simulink model "MovimientoArmonicoAmortiguado"  (R2024b)
settings: Solver=ode4  StartTime=0.0  StopTime=100.0  FixedStep=0.01  RelTol=1e-3
settings Model: Creator=Miguel  LastModifiedBy=Miguel

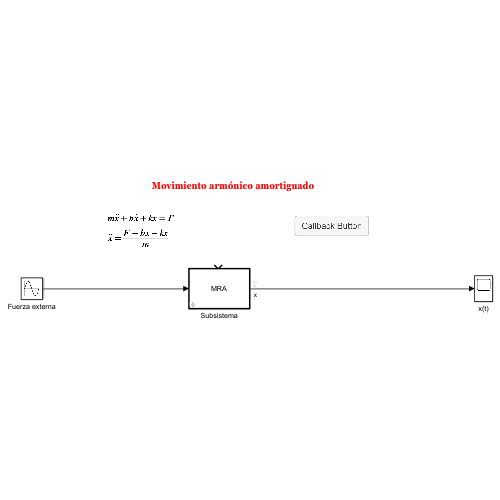
[thumbnail: Simulink's stored preview of the top-level diagram]
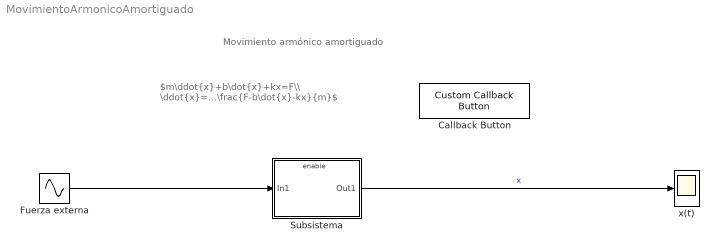
== system MovimientoArmonicoAmortiguado ==
  note: $m\ddot{x}+b\dot{x}+kx=F\\ \ddot{x}=\frac{F-b\dot{x}-kx}{m}$
  note: Movimiento armónico amortiguado
  Callback Button : CustomCallbackButton  Configuration="{\"components\":[{\"name\":\"BackgroundImageComponent\",\"settings\":{\"image\":{\"size\":[0,0],\"src\":\"default\",\"srcOrientation\":\"Right\"},\"position\":[0,0,1,1]}},{\"name\":\"ButtonStateComponent\",\"settings\":{\"buttonType\":\"momentary\",\"clickFcn\":\"close all\\nx = out.posicion;\\nv = out.velocidad;\\nn = length(x(1,:));\\n\\nplot(x(:,2),v(:,2),'LineWidth',3)\\nhold on\\n\\nfor k=3:n\\n    plot(x(:,k),v(:,k),'LineWidth',3)\\nend\\n\\nxlabel('$x$','Interpreter','latex','FontSize',14)\\nxlabel('$\\\\dot{x}$','Interpreter','latex','FontSize',14)\\ngrid on\\nhold off\",\"onValue\":1,\"position\":[0,0,1,1],\"pressDelay\":\"500\",\"pressFcn\":\"\",\"repeatInterval\":\"0\",\"states\":[{\"horizontalAlignment\":\"center\",\"image\":{\"position\":[0,0,1,1],\"size\":[1,1],\"src\":\"default\",\"srcOrientation\":\"Right\"},\"label\":{\"color\":[0.01176470588,0.01176470588,0.01176470588,1],\"icon\":{\"size\":[0,0],\"src\":\"default\",\"srcOrientation\":\"Right\"},\"iconOffset\":0,\"iconPlacement\":\"left\",\"opacity\":1,\"show\":true,\"text\":{\"content\":\"Callback Button\",\"font\":\"Helvetica\"}},\"labelOffset\":[0,0],\"verticalAlignment\":\"middle\"},{\"horizontalAlignment\":\"center\",\"image\":{\"position\":[0,0,1,1],\"size\":[1,1],\"src\":\"default\",\"srcOrientation\":\"Right\"},\"label\":{\"color\":[0.01176470588,0.01176470588,0.01176470588,1],\"icon\":{\"size\":[0,0],\"src\":\"default\",\"srcOrientation\":\"Right\"},\"iconOffset\":0,\"iconPlacement\":\"left\",\"opacity\":1,\"show\":true,\"text\":{\"content\":\"Callback Button\",\"font\":\"Helvetica\"}},\"labelOffset\":[0,0],\"verticalAlignment\":\"middle\"},{\"horizontalAlignment\":\"center\",\"image\":{\"position\":[0,0,1,1],\"size\":[1,1],\"src\":\"default\",\"srcOrientation\":\"Right\"},\"label\":{\"color\":[0.01176470588,0.01176470588,0.01176470588,1],\"icon\":{\"size\":[0,0],\"src\":\"default\",\"srcOrientation\":\"Right\"},\"iconOffset\":0,\"iconPlacement\":\"left\",\"opacity\":1,\"show\":true,\"text\":{\"content\":\"Callback Button\",\"font\":\"Helvetica\"}},\"labelOffset\":[0,0],\"verticalAlignment\":\"middle\"},{\"horizontalAlignment\":\"center\",\"image\":{\"position\":[0,0,1,1],\"size\":[1,1],\"src\":\"default\",\"srcOrientation\":\"Right\"},\"label\":{\"color\":[0.01176470588,0.01176470588,0.01176470588,1],\"icon\":{\"size\":[0,0],\"src\":\"default\",\"srcOrientation\":\"Right\"},\"iconOffset\":0,\"iconPlacement\":\"left\",\"opacity\":1,\"show\":true,\"text\":{\"content\":\"Callback Button\",\"font\":\"Helvetica\"}},\"labelOffset\":[0,0],\"verticalAlignment\":\"middle\"}]}},{\"name\":\"ForegroundImageComponent\",\"settings\":{\"image\":{\"size\":[0,0],\"src\":\"default\",\"srcOrientation\":\"Right\"},\"isForeground\":1,\"position\":[0,0,1,1]}}],\"settings\":{\"BindingType\":\"standalone\",\"backgroundColor\":[244,244,244,1],\"backgroundOffset\":0.2,\"backgroundOpacity\":1,\"fixedAspectRatio\":\"off\",\"foregroundColor\":[0.01176470588,0.01176470588,0.01176470588,1],\"migratedFromLegacy\":true,\"useBackgroundColor\":true,\"variant\":\"callback\",\"version\":\"R2023a\"},\"type\":\"Button\"}"  CustomBackgroundColor="{\"color\":[0.9568627451,0.9568627451,0.9568627451],\"show\":true}"
  Fuerza externa : Sin  Amplitude=0  Frequency=1/(2*pi)  SampleTime=0
  Subsistema : Subsystem  mask{m=1, k=1, b=0.25}
      mask prompts: m "masa"; k "resorte"; b "amortiguador"
      mask Display: disp('MRA')
  x(t) : Scope
  wires:
  Subsistema/1(Out1) -> x(t)/1  "x"
  Fuerza externa/1 -> Subsistema/1(In1)

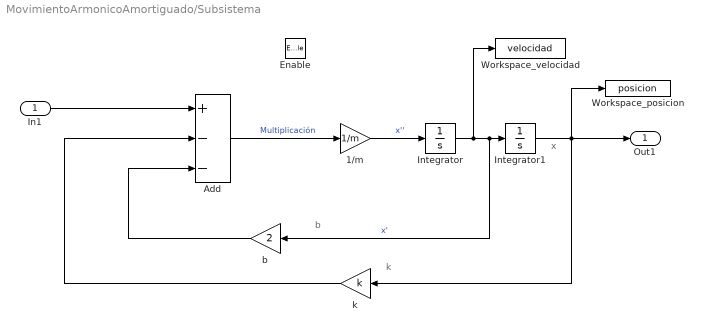
== system MovimientoArmonicoAmortiguado/Subsistema ==
  note: k
  note: b
  note: x
  In1 : Inport
  Enable : EnablePort
  1/m : Gain  Gain=1/m
  Add : Sum  Inputs=+--
  Integrator : Integrator
  Integrator1 : Integrator  InitialCondition=linspace(-1,1,20)
  Workspace_posicion : ToWorkspace  VariableName=posicion  SampleTime=-1
  Workspace_velocidad : ToWorkspace  VariableName=velocidad  SampleTime=-1
  b : Gain  Gain=2
  k : Gain  Gain=k
  Out1 : Outport
  wires:
  Integrator/1 -> b/1, Integrator1/1, Workspace_velocidad/1  "x'"
  Add/1 -> 1/m/1  "Multiplicación"
  1/m/1 -> Integrator/1  "x''"
  k/1 -> Add/2
  Integrator1/1 -> Workspace_posicion/1, Out1/1, k/1
  b/1 -> Add/3
  In1/1 -> Add/1
